simulink model "sm"  (R2018a)
settings: Solver=VariableStepAuto  StartTime=0.0  StopTime=60  MaxStep=1e-2  RelTol=1e-3
undefined symbols (not defined in the file): Am, b, Bm, Cm, Dm, k1, k2, k3, m1, m2
settings Model: Creator=carma  LastModifiedBy=carma

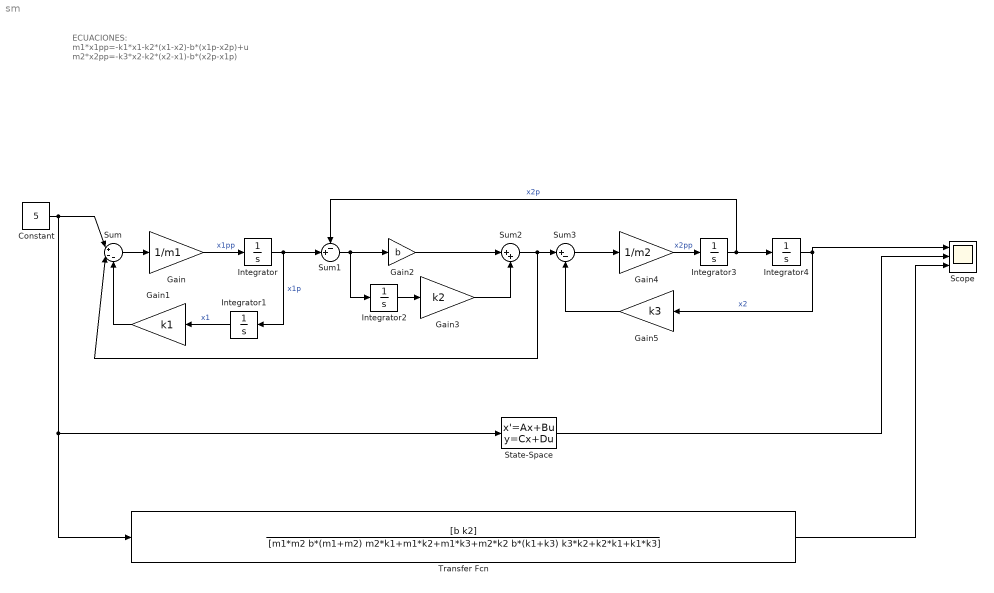
== system sm ==
  note: ECUACIONES:
      | m1*x1pp=-k1*x1-k2*(x1-x2)-b*(x1p-x2p)+u
      | m2*x2pp=-k3*x2-k2*(x2-x1)-b*(x2p-x1p)
  Constant : Constant  Value=5
  Gain : Gain  Gain=1/m1
  Gain1 : Gain  Gain=k1
  Gain2 : Gain  Gain=b
  Gain3 : Gain  Gain=k2
  Gain4 : Gain  Gain=1/m2
  Gain5 : Gain  Gain=k3
  Integrator{,1..4} (5 alike) : Integrator
  Scope : Scope  NumInputPorts=3
  State-Space : StateSpace  A=Am  B=Bm  C=Cm  D=Dm  InitialCondition=0
  Sum : Sum  Inputs=|+--
  Sum1 : Sum  Inputs=-+|
  Sum2 : Sum  Inputs=|++
  Sum3 : Sum  Inputs=|+-
  Transfer Fcn : TransferFcn  Numerator=[b k2]  Denominator=[m1*m2 b*(m1+m2) m2*k1+m1*k2+m1*k3+m2*k2 b*(k1+k3) k3*k2+k2*k1+k1*k3]
  wires:
  Gain/1 -> Integrator/1  "x1pp"
  Sum/1 -> Gain/1
  Integrator1/1 -> Gain1/1  "x1"
  Gain1/1 -> Sum/3
  Integrator/1 -> Sum1/2, Integrator1/1  "x1p"
  Sum1/1 -> Integrator2/1, Gain2/1
  Gain2/1 -> Sum2/1
  Integrator2/1 -> Gain3/1
  Gain3/1 -> Sum2/2
  Gain4/1 -> Integrator3/1  "x2pp"
  Sum2/1 -> Sum/2, Sum3/1
  Sum3/1 -> Gain4/1
  Gain5/1 -> Sum3/2
  Integrator3/1 -> Sum1/1, Integrator4/1  "x2p"
  Integrator4/1 -> Scope/1, Gain5/1  "x2"
  Constant/1 -> Transfer Fcn/1, State-Space/1, Sum/1
  State-Space/1 -> Scope/2
  Transfer Fcn/1 -> Scope/3
